simulink model "RoboticFish_NGC"  (R2020b)
settings: Solver=ode4  StartTime=0.0  StopTime=120  FixedStep=0.00025  RelTol=1e-3  EnableMultiTasking=on
undefined symbols (not defined in the file or in its folder): sigbuilder_block
undefined symbols (not defined in the file): Ref, uCMD
libraries: sharedutil x11, pid_lib x5, dspsigops x2, dspmtrx3 x1, vrlib x1
(part 1 of 2)
settings Model: Creator=Waqas Ali Waqar  LastModifiedBy=Waqas Ali Waqar
settings SolverCC: ConcurrentTasks=on  AutoInsertRateTranBlk=on  InsertRTBMode=Never (minimum delay)
settings DataIOCC: SaveFormat=StructureWithTime
settings OptimizationCC: BlockReduction=off  OptimizeBlockIOStorage=off  BufferReuse=off  GlobalBufferReuse=off  ExpressionFolding=off  PassReuseOutputArgsThreshold=0  LocalBlockOutputs=off  OptimizeBlockOrder=speed  OptimizeDataStoreBuffers=off  BusAssignmentInplaceUpdate=off
settings DebuggingCC: ParameterTunabilityLossMsg=error
settings HardwareCC: ProdBitPerPointer=32  ProdBitPerSizeT=32  ProdBitPerPtrDiffT=32  ProdLargestAtomicFloat=None  ProdWordSize=32  ProdLongLongMode=on  ProdHWDeviceType=Generic->32-bit x86 compatible
settings SFSimCC: MATLABDynamicMemAlloc=off  CustomCodeUndefinedFunction=UseInterfaceOnly
settings RTWCC: GenerateReport=on  RTWVerbose=off  LaunchReport=on  RTWCompilerOptimization=on
settings CodeAppCC: ForceParamTrailComments=on  OperatorAnnotations=on
settings GRTTargetCC: TargetLangStandard=C89/C90 (ANSI)

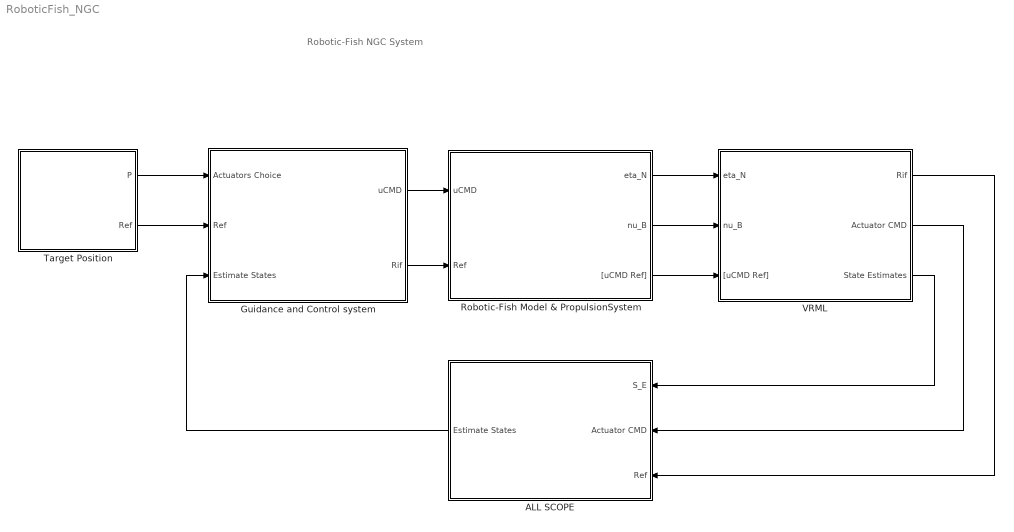
== system RoboticFish_NGC ==
  note: Robotic-Fish NGC System
  ALL SCOPE : Subsystem
  Guidance and Control system : Subsystem
  Robotic-Fish Model & PropulsionSystem : Subsystem  mask{Ig=[0.0268 0 0;0 0.0512 0;0 0 0.043], m=3.259, rho=1000, R=0.05, L=0.55, cdf=0.5, cdt=1, W=32.59, B=32.59, rG_B=[0;0;0], rB_B=[0;0;-0.02], DL=diag([0;0;0;0;0;0]), c=0.14, S=0.014, Theta0deg=15, a2=3.60, a1=-0.026, a0=-0.163, b2=8.952, b1=-0.359, b0=0.012, c2=51.81, d2=33.01, phisurge=0.59, phisway=0.44, phiyaw=0.53, cL=2, xfin=0.11, yfin=0.11, zfin=0.75, Max_Delta=45, Min_Delta=-45, Sfin=0.017, HT1Max=1.12, e1=[1;0;0], r1=[0;-0.11;0], HT2Max=1.12, e2=[1;0;0], r2=[0;0.11;0], VT1Max=1.12, e3=[0;0;1], r3=[0;0;-0.03]}
      mask prompts: Ig "Inertia Tensor Ig:"; m "Mass m:"; rho "Seawater Density rho:"; R "Body Radius R:"; L "Body Lenght L:"; cdf "Drag Weight cdf:"; cdt "Drag Weight cdt [0.8-1.2]:"; W "Weight"; B "Buoyancy"; DL "Linear Damping Matrix"; c "c-Foil Mean Chord (m)"; S "S-Foil area (m^2)"; Theta0deg "Theta0-Oscillation amplitude"; cL "fin lift coefficient  cL:"; xfin "fin axial position xfin:"; yfin "fin axial position yfin:"; zfin "fin axial position zfin:"; Max_Delta "Max fin rotation angle"; Min_Delta "Min fin rotation angle"; Sfin "fin platform area Sfin:"; HT1Max "Max Thrust (HT1):"; e1 "e1 (HT1):"; r1 "r1 (HT1):"; HT2Max "Max Thrust (HT2):"; e2 "e2 (HT2 ):"; r2 "r2 (HT2):"; VT1Max "Max Thrust (VT1):"; e3 "e3 (VT1):"; r3 "r3 (VT1):"
      mask init:
      | %%%%%%%%%%%%%%%%%%%%%%%%%%%%%%%%%%%%%%%%%%%%%%%%%%%%%%%
      | %%%%%%%%%%%%%%%%%%%  DINAMICA  %%%%%%%%%%%%%%%%%%%%%%%%
      | %%%%%%%%%%%%%%%%%%%%%%%%%%%%%%%%%%%%%%%%%%%%%%%%%%%%%%%
      | 
      | % Matrice di inerzia del corpo rigido
      | Ib = Ig-m*skewsymm(rG_B)*skewsymm(rG_B);
      | MRB = [m*eye(3,3) -m*skewsymm(rG_B); m*skewsymm(rG_B) Ib];
      | 
      | %Masse aggiunte
      | X_udot = 0.1*m;
      | Y_vdot = pi*rho*R^2*L;
      | Z_wdot = pi*rho*R^2*L;
      | K_pdot = 0;
      | M_qdot = (pi*rho*R^2*L^3)/12;
      | N_rdot = (pi*rho*R^2*L^3)/12;
      | 
      | %Matrice delle masse aggiunte
      | MA = diag([X_udot;Y_vdot;Z_wdot;K_pdot;M_qdot;N_rdot]);
      | 
      | %Matrice di inerzia (incluse le masse aggiunte)
      | M = MRB + MA;
      | inv_M = inv(M);
      | M11 = MA(1:3,1:3);    M12 = MA(1:3,4:6);
      | M21 = MA(4:6,1:3);    M22 = MA(4:6,4:6);
      | 
      | %%Attrito viscoso
      | 
      | %Aree
      | Af = pi*R^2;
      | At = 2*pi*R;
      | 
      | %Coefficienti
      | X_uu = 2*rho*Af*cdf/2;
      | Y_vv = rho*At*cdt/2;
      | Z_ww = rho*At*cdt/2;
      | K_pp = (rho*At*cdt*L^3)/16;
      | M_qq = (rho*At*cdt*L^3)/16;
      | N_rr = (rho*At*cdt*L^3)/16;
      | 
      | dQ = ([X_uu;Y_vv;Z_ww;K_pp;M_qq;N_rr]);
      | 
      | 
      | %%%%%%%%%%%%%%%%%%%%%%%%%%%%%%%%%%%%%%%%%%%%%%%%%%%%%%%
      | %%%%%%%%%%%%%%%%%%%  PROP HT3  %%%%%%%%%%%%%%%%%%%%%%%%
      | %%%%%%%%%%%%%%%%%%%%%%%%%%%%%%%%%%%%%%%%%%%%%%%%%%%%%%%
      | 
      | Theta0=Theta0deg*pi/180
      | TanTheta0=tan(Theta0)
      | 
      | 
      | %%%%%%%%%%%%%%%%%%%%%%%%%%%%%%%%%%%%%%%%%%%%%%%%%%%%%%%
      | %%%%%%%%%%%%%%%%%%%  PROP HT1 HT2 VT1  %%%%%%%%%%%%%%%%
      | %%%%%%%%%%%%%%%%%%%%%%%%%%%%%%%%%%%%%%%%%%%%%%%%%%%%%%%
      | 
      | K1 = HT1Max*9.81;
      | K2 = HT2Max*9.81;
      | K3 = VT1Max*9.81;
      | HT_prop = [e1 e2;skewsymm(r1)*e1 skewsymm(r2)*e2]*diag([K1;K2]);
      | VT_prop = [e3 ;skewsymm(r3)*e3 ]*K3;
      | 
      | 
      | %%%%%%%%%%%%%%%%%%%%%%%%%%%%%%%%%%%%%%%%%%%%%%%%%%%%%%%
      | %%%%%%%%%%%%%%%%%%%  PROP VT1 VT2  %%%%%%%%%%%%%%%%%%%%
      | %%%%%%%%%%%%%%%%%%%%%%%%%%%%%%%%%%%%%%%%%%%%%%%%%%%%%%%
      | 
      | Max_Delta_rad=Max_Delta*pi/180;
      | Min_Delta_rad=Min_Delta*pi/180;
      mask DialogControl DescGroupVar Prompt: Robotic Fish Paramteres
      mask DialogControl Container14 Prompt: Robotic Fish Parameters
      mask DialogControl Container17 Prompt: Caudal Fin Parameters
      mask DialogControl Container18 Prompt: Pectoral Fins Parameters
      mask DialogControl Container19 Prompt: Thrusters Parameters
  Target Position : Subsystem  mask{PC=Normal, SP=Way-Points based Path, Xr=0, Yr=0, Zr=0}
      mask init:
      | if (SP == 1)
      |     Flag=0;
      | end
      | if (SP == 2)
      |     Flag=1;
      | end
      | 
      | if (PC == 1)
      |     PropChoice=0;
      | end
      | if (PC == 2)
      |     PropChoice=1;
      | end
      mask TypeOptions PC: Normal | Only Propeller
      mask TypeOptions SP: Way-Points based Path | Way-Point Position
      mask DialogControl DescGroupVar Prompt: Target Position
      mask DialogControl Container8 Prompt: Actuator Choice
      mask DialogControl Container7 Prompt: Select Target
      mask DialogControl Container9 Prompt: Way-Point position
  "VRML " : Subsystem
  wires:
  Robotic-Fish Model & PropulsionSystem/2(nu_B) -> "VRML "/2(nu_B)
  Target Position/1(P) -> Guidance and Control system/1(Actuators Choice)
  Robotic-Fish Model & PropulsionSystem/1(eta_N) -> "VRML "/1(eta_N)
  Target Position/2(Ref) -> Guidance and Control system/2(Ref)
  ALL SCOPE/1(Estimate States) -> Guidance and Control system/3(Estimate States)
  "VRML "/3(State Estimates) -> ALL SCOPE/1(S_E)
  "VRML "/2(Actuator CMD) -> ALL SCOPE/2(Actuator CMD)
  "VRML "/1(Rif) -> ALL SCOPE/3(Ref)
  Robotic-Fish Model & PropulsionSystem/3("[uCMD Ref]") -> "VRML "/3("[uCMD Ref]")
  Guidance and Control system/1(uCMD) -> Robotic-Fish Model & PropulsionSystem/1(uCMD)
  Guidance and Control system/2(Rif) -> Robotic-Fish Model & PropulsionSystem/2(Ref)

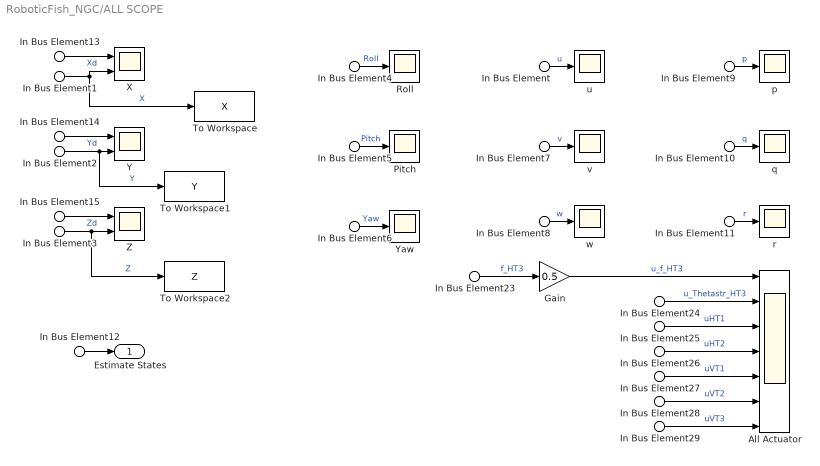
== system RoboticFish_NGC/ALL SCOPE ==
  In Bus Element12 : Inport  PortName=S_E
  In Bus Element2 : Inport  PortName=S_E  Element=Position.Y
  In Bus Element3 : Inport  PortName=S_E  Element=Position.Z
  In Bus Element4 : Inport  PortName=S_E  Element=Position.Roll
  In Bus Element5 : Inport  PortName=S_E  Element=Position.Pitch
  In Bus Element6 : Inport  PortName=S_E  Element=Position.Yaw
  In Bus Element1 : Inport  PortName=S_E  Element=Position.X
  In Bus Element : Inport  PortName=S_E  Element=Velocity.u
  In Bus Element7 : Inport  PortName=S_E  Element=Velocity.v
  In Bus Element8 : Inport  PortName=S_E  Element=Velocity.w
  In Bus Element9 : Inport  PortName=S_E  Element=Velocity.p
  In Bus Element10 : Inport  PortName=S_E  Element=Velocity.q
  In Bus Element11 : Inport  PortName=S_E  Element=Velocity.r
  In Bus Element23 : Inport  Port=2  PortName=Actuator CMD  Element=f_HT3
  In Bus Element24 : Inport  Port=2  PortName=Actuator CMD  Element=Thetastr_HT3
  In Bus Element25 : Inport  Port=2  PortName=Actuator CMD  Element=uHT1
  In Bus Element26 : Inport  Port=2  PortName=Actuator CMD  Element=uHT2
  In Bus Element27 : Inport  Port=2  PortName=Actuator CMD  Element=uVT1
  In Bus Element28 : Inport  Port=2  PortName=Actuator CMD  Element=D_VT2
  In Bus Element29 : Inport  Port=2  PortName=Actuator CMD  Element=D_VT3
  In Bus Element13 : Inport  Port=3  PortName=Ref  Element=Xr
  In Bus Element14 : Inport  Port=3  PortName=Ref  Element=Yr
  In Bus Element15 : Inport  Port=3  PortName=Ref  Element=Zr
  All Actuator : Scope  NumInputPorts=7
  Gain : Gain  Gain=0.5
  Pitch : Scope
  Roll : Scope
  To Workspace : ToWorkspace  VariableName=X  SampleTime=0.25
  To Workspace1 : ToWorkspace  VariableName=Y  SampleTime=0.25
  To Workspace2 : ToWorkspace  VariableName=Z  SampleTime=0.25
  X : Scope  NumInputPorts=2
  Y : Scope  NumInputPorts=2
  Yaw : Scope
  Z : Scope  NumInputPorts=2
  p : Scope
  q : Scope
  r : Scope
  u : Scope
  v : Scope
  w : Scope
  Estimate States : Outport  VectorParamsAs1DForOutWhenUnconnected=off
  wires:
  In Bus Element4/1 -> Roll/1  "Roll"
  In Bus Element5/1 -> Pitch/1  "Pitch"
  In Bus Element6/1 -> Yaw/1  "Yaw"
  In Bus Element/1 -> u/1  "u"
  In Bus Element7/1 -> v/1  "v"
  In Bus Element8/1 -> w/1  "w"
  In Bus Element9/1 -> p/1  "p"
  In Bus Element10/1 -> q/1  "q"
  In Bus Element11/1 -> r/1  "r"
  In Bus Element12/1 -> Estimate States/1
  In Bus Element15/1 -> Z/1  "Zd"
  In Bus Element3/1 -> To Workspace2/1, Z/2  "Z"
  In Bus Element2/1 -> To Workspace1/1, Y/2  "Y"
  In Bus Element14/1 -> Y/1  "Yd"
  In Bus Element23/1 -> Gain/1  "f_HT3"
  In Bus Element24/1 -> All Actuator/2  "u_Thetastr_HT3"
  In Bus Element25/1 -> All Actuator/3  "uHT1"
  In Bus Element26/1 -> All Actuator/4  "uHT2"
  In Bus Element27/1 -> All Actuator/5  "uVT1"
  In Bus Element28/1 -> All Actuator/6  "uVT2"
  In Bus Element29/1 -> All Actuator/7  "uVT3"
  Gain/1 -> All Actuator/1  "u_f_HT3"
  In Bus Element1/1 -> To Workspace/1, X/2  "X"
  In Bus Element13/1 -> X/1  "Xd"

== system RoboticFish_NGC/Guidance and Control system ==
  Actuators Choice : Inport
  Ref : Inport  Port=2
  Estimate States : Inport  Port=3
  " Control system" : Subsystem
  " Guidance system" : Subsystem
  uCMD : Outport  VectorParamsAs1DForOutWhenUnconnected=off
  Rif : Outport  Port=2  VectorParamsAs1DForOutWhenUnconnected=off
  wires:
  Estimate States/1 -> " Guidance system"/2(Estimate States I)
  Ref/1 -> Rif/1, " Guidance system"/1(Ref)
  " Guidance system"/1("LOS ") -> " Control system"/1(LOS)
  Actuators Choice/1 -> " Control system"/2(Actuators Choice)
  " Guidance system"/2(Estimate States O) -> " Control system"/3(Estimate states)
  " Control system"/1(uCMD) -> uCMD/1

== system RoboticFish_NGC/Robotic-Fish Model & PropulsionSystem ==
  uCMD : Inport
  In Bus Element1 : Inport  Port=2  PortName=Ref
  Bus Creator : BusCreator  Inputs=2
  Memory : Memory
  Propulsion System : Subsystem
  RF Dynamics and Kinematics (Attitude rappresentation: Quaternions) : Subsystem
      mask Display: image('C:\Users\Waqas Ali Waqar\Desktop\Robotic_Fish_Simulink\Robotic_Fish_Simulink\Imm\RF.png');
  eta_N : Outport  VectorParamsAs1DForOutWhenUnconnected=off
  nu_B : Outport  Port=2  VectorParamsAs1DForOutWhenUnconnected=off
  "[uCMD Ref]" : Outport  Port=3  VectorParamsAs1DForOutWhenUnconnected=off
  wires:
  RF Dynamics and Kinematics (Attitude rappresentation: Quaternions)/1(nu_B) -> nu_B/1, Memory/1  "[u    v    w    p    q    r]"
  Memory/1 -> Propulsion System/1(nu_B)
  RF Dynamics and Kinematics (Attitude rappresentation: Quaternions)/2(eta_N) -> eta_N/1  "[x   y   z  q0  q1  q2  q3]"
  uCMD/1 -> Propulsion System/2(uCMD)
  Propulsion System/2(ucmd) -> Bus Creator/1  "uCMD"
  Propulsion System/1(Tau_B) -> RF Dynamics and Kinematics (Attitude rappresentation: Quaternions)/1(tau_B)  "[Tau_X, Tau_Y, Tau_Z, Tau_Roll, Tau_Pitch, Tau_Yaw]"
  In Bus Element1/1 -> Bus Creator/2  "Ref"
  Bus Creator/1 -> "[uCMD Ref]"/1

== system RoboticFish_NGC/Target Position ==
  "  " : Subsystem  Tag=STV Subsys  LoadFcn=sigbuilder_block('load');  StartFcn=sigbuilder_block('start');  StopFcn=sigbuilder_block('stop');  ClipboardFcn=sigbuilder_block('clipboard');  mask(Sigbuilder block){tuvar=[0:10]}
      mask help: Simulink:masks:SigbuilderBlock_MD
      mask init:
      | if ~strcmp(get_param(bdroot(gcbh),'SimulationStatus'),'stopped') tuvar = sigbuilder_block('maskInit'); end
      settings: CopyFcn=sigbuilder_block('copy');  DeleteFcn=sigbuilder_block('delete');  ModelCloseFcn=sigbuilder_block('modelClose');  PreSaveFcn=sigbuilder_block('preSave');  PauseFcn=sigbuilder_block('pause');  ContinueFcn=sigbuilder_block('continue');  NameChangeFcn=sigbuilder_block('namechange');  OpenFcn=sigbuilder_block('open',[6 30 1012.5 447.75 ]);  CloseFcn=sigbuilder_block('close');
      mask Display: plot(0, 0, 100, 100,[2, 2, 32, 32, 2], [68, 8, 8, 68, 68],[32, 2], [38, 38], [32, 19, 2],[53, 60, 44], [32, 17, 17, 2],[16, 16, 31, 31]);txt = getActiveGroup(gcbh);text(2, 100, txt,'verticalAlignment', 'top');
  Bus Creator : BusCreator  Inputs=3
  Bus Creator1 : BusCreator  Inputs=3
  Constant : Constant  Value=Flag
  Constant1 : Constant  Value=Xr
  Constant2 : Constant  Value=Yr
  Constant3 : Constant  Value=Zr
  Constant4 : Constant  Value=PropChoice
  Switch : Switch  Criteria=u2 > Threshold
  Bus Element Out : Outport  VectorParamsAs1DForOutWhenUnconnected=off  PortName=P  Element=Actuators Choice
  Ref : Outport  Port=2  VectorParamsAs1DForOutWhenUnconnected=off
  wires:
  "  "/3(Zr) -> Bus Creator1/3  "Zr"
  Constant/1 -> Switch/2
  Bus Creator1/1 -> Switch/3
  Bus Creator/1 -> Switch/1
  Switch/1 -> Ref/1
  Constant3/1 -> Bus Creator/3  "Zr"
  Constant2/1 -> Bus Creator/2  "Yr"
  Constant1/1 -> Bus Creator/1  "Xr"
  Constant4/1 -> Bus Element Out/1  "PCHOICE"
  "  "/2(Yr) -> Bus Creator1/2  "Yr"
  "  "/1(Xr) -> Bus Creator1/1  "Xr"

== system RoboticFish_NGC/VRML  ==
  eta_N : Inport
  nu_B : Inport  Port=2
  In Bus Element1 : Inport  Port=3  PortName=[uCMD Ref]  Element=uCMD
  In Bus Element : Inport  Port=3  PortName=[uCMD Ref]  Element=Ref
  In Bus Element2 : Inport  Port=3  PortName=[uCMD Ref]  Element=Ref
  Bus Selector : BusSelector  OutputSignals=uVT3,uVT2,uHT3,uVT1,uHT2,uHT1
  Estimate States : Subsystem
  RF Position and Rotation to VR Translation and Rotation : Subsystem
  RF Virtual Reality Display : vrlib/VR Sink  InstantiateOnLoad=on  SampleTime=0.1  ViewEnable=on  RemoteChange=off  RemoteView=off  FieldsWritten=WayPoint.rotation.4.1.1.double#WayPoint.translation.3.1.1.double#RF.rotation.4.1.1.double#RF.translation.3.1.1.double#VT3.rotation.4.1.1.double#Vt2.rotation.4.1.1.double#HT3.rotation.4.1.1.double#VT1.rotation.4.1.1.double#HT2.rotation.4.1.1.double#HT1.rotation.4.1.1.double#ViewPoints.translation.3.1.1.double  WorldFileName=Final_RF.wrl  AutoView=on  VideoDimensions=[]  AllowVariableSize=off  FigureProperties="{'Position', 'Name', 'Viewpoint', 'CameraBound', 'CameraDirection', 'CameraPosition', 'CameraUpVector', 'ZoomFactor', 'Antialiasing', 'Headlight', 'Lighting', 'NavPanel', 'Sound', 'StatusBar', 'Stereo3D', 'Stereo3DCameraOffset', 'Stereo3DHIT', 'ToolBar', 'Textures', 'Transparency', 'Triad', 'Wireframe', 'NavZones', 'NavMode', 'NavSpeed', 'CaptureFileFormat', 'CaptureFileName', 'Record2DCompressMethod', 'Record2DCompressQuality', 'Record2D', 'Record2DFileName', 'Record2DFPS'; [5.0000000000000000e+00   1.2200000000000000e+02   5.7600000000000000e+02   3.2000000000000000e+02], '', 'RF_UP_CAMERA', 'on', [0.0000000000000000e+00   0.0000000000000000e+00  -1.0000000000000000e+00], [0.0000000000000000e+00   0.0000000000000000e+00   0.0000000000000000e+00], [0.0000000000000000e+00   1.0000000000000000e+00   0.0000000000000000e+00], [1.0000000000000000e+00], 'on', 'on', 'on', 'halfbar', 'on', 'on', 'off', [1.0000000149011612e-01], [0.0000000000000000e+00], 'on', 'on', 'on', 'none', 'off', 'off', 'fly', 'normal', 'tif', '%f_anim_%n.tif', 'auto', [7.5000000000000000e+01], 'off', '%f_anim_%n.avi', 'auto'}"
  Thruster rotation : Subsystem
  WayPoint Position and Rotation To VR Translation and Rotation : Subsystem
  Rif : Outport  VectorParamsAs1DForOutWhenUnconnected=off
  Actuator CMD : Outport  Port=2  VectorParamsAs1DForOutWhenUnconnected=off
  State Estimates : Outport  Port=3  VectorParamsAs1DForOutWhenUnconnected=off
  wires:
  eta_N/1 -> Estimate States/2(eta), RF Position and Rotation to VR Translation and Rotation/1(eta_N)
  nu_B/1 -> Estimate States/1(nu)
  RF Position and Rotation to VR Translation and Rotation/1(VR Rotation) -> WayPoint Position and Rotation To VR Translation and Rotation/2(RF VR Rotation), RF Virtual Reality Display/3
  Estimate States/1(Estimate States) -> State Estimates/1
  In Bus Element2/1 -> WayPoint Position and Rotation To VR Translation and Rotation/1(Waypoint Position)
  Thruster rotation/1(T_rotation) -> Bus Selector/1
  In Bus Element1/1 -> Actuator CMD/1, Thruster rotation/1(uCMD)
  In Bus Element/1 -> Rif/1
  WayPoint Position and Rotation To VR Translation and Rotation/2(Waypoint VR Translation) -> RF Virtual Reality Display/2
  WayPoint Position and Rotation To VR Translation and Rotation/1(Waypoint VR Rotation) -> RF Virtual Reality Display/1
  Bus Selector/1 -> RF Virtual Reality Display/5  "<uVT3>"
  Bus Selector/2 -> RF Virtual Reality Display/6  "<uVT2>"
  Bus Selector/3 -> RF Virtual Reality Display/7  "<uHT3>"
  Bus Selector/4 -> RF Virtual Reality Display/8  "<uVT1>"
  Bus Selector/5 -> RF Virtual Reality Display/9  "<uHT2>"
  Bus Selector/6 -> RF Virtual Reality Display/10  "<uHT1>"
  RF Position and Rotation to VR Translation and Rotation/2(VR Translation) -> RF Virtual Reality Display/11, RF Virtual Reality Display/4

== system RoboticFish_NGC/Guidance and Control system/ Control system ==
  LOS : Inport
  Actuators Choice : Inport  Port=2
  Estimate states : Inport  Port=3
  Control Allocator : Subsystem
  Control Law : Subsystem
  uCMD : Outport  VectorParamsAs1DForOutWhenUnconnected=off
  wires:
  Control Law/1(Tin) -> Control Allocator/1(Tin)
  LOS/1 -> Control Law/1(LOS)
  Estimate states/1 -> Control Law/2(Estimate States)
  Control Law/2(Actuators Choice O) -> Control Allocator/2(Actuators Choice)
  Control Allocator/1(uCMD) -> uCMD/1
  Actuators Choice/1 -> Control Law/3(P)

== system RoboticFish_NGC/Guidance and Control system/ Guidance system ==
  In Bus Element9 : Inport  PortName=Ref  Element=Xr
  In Bus Element10 : Inport  PortName=Ref  Element=Yr
  In Bus Element8 : Inport  PortName=Ref  Element=Zr
  In Bus Element3 : Inport  Port=2  PortName=Estimate States I
  In Bus Element4 : Inport  Port=2  PortName=Estimate States I  Element=Position.X
  In Bus Element5 : Inport  Port=2  PortName=Estimate States I  Element=Position.Y
  In Bus Element6 : Inport  Port=2  PortName=Estimate States I  Element=Position.Z
  Bus Creator : BusCreator  Inputs=3
  Distance : Subsystem
  LOS law : Subsystem
  Mux1 : Mux  Inputs=3
  Mux4 : Mux  Inputs=3
  Selector : Selector  InputPortWidth=3  IndexOptions=Index vector (dialog)  Indices=[3]  OutputSizes=1
  Selector1 : Selector  InputPortWidth=3  IndexOptions=Index vector (dialog)  Indices=[1 2]  OutputSizes=1
  Selector2 : Selector  InputPortWidth=3  IndexOptions=Index vector (dialog)  Indices=[1 2]  OutputSizes=1
  Sum2 : Sum  Inputs=|+-
  "LOS " : Outport  VectorParamsAs1DForOutWhenUnconnected=off
  Estimate States O : Outport  Port=2  VectorParamsAs1DForOutWhenUnconnected=off
  wires:
  In Bus Element3/1 -> Estimate States O/1
  In Bus Element4/1 -> Mux1/1
  In Bus Element5/1 -> Mux1/2
  LOS law/1(Yaw_d) -> Bus Creator/2  "Yaw_d"
  Selector/1 -> Bus Creator/3  "Ze"
  Bus Creator/1 -> "LOS "/1
  Sum2/1 -> Selector1/1, Selector/1, Selector2/1  "[Xe Ye Ze]"
  Distance/1(D) -> Bus Creator/1  "D"
  In Bus Element9/1 -> Mux4/1
  In Bus Element10/1 -> Mux4/2
  Mux4/1 -> Sum2/1  "[Xr Yr Zr]"
  Mux1/1 -> Sum2/2  "[X Y Z]"
  Selector1/1 -> Distance/1("[Xe Ye]")  "[Xe Ye]"
  Selector2/1 -> LOS law/1("[Xe Ye]")  "[Xe Ye]"
  In Bus Element6/1 -> Mux1/3
  In Bus Element8/1 -> Mux4/3

== system RoboticFish_NGC/Robotic-Fish Model & PropulsionSystem/Propulsion System ==
  nu_B : Inport
  In Bus Element : Inport  Port=2  PortName=uCMD
  In Bus Element1 : Inport  Port=2  PortName=uCMD  Element=f_HT3
  In Bus Element4 : Inport  Port=2  PortName=uCMD  Element=uHT2
  In Bus Element5 : Inport  Port=2  PortName=uCMD  Element=uVT1
  In Bus Element6 : Inport  Port=2  PortName=uCMD  Element=uVT2
  In Bus Element7 : Inport  Port=2  PortName=uCMD  Element=uVT3
  In Bus Element8 : Inport  Port=2  PortName=uCMD  Element=Thetastr_HT3
  In Bus Element2 : Inport  Port=2  PortName=uCMD  Element=uHT1
  Bus Creator : BusCreator  Inputs=2
  Bus Creator1 : BusCreator  Inputs=2
  Horizontal Force and Moment (Tau_H) : Subsystem
  Subsystem : Subsystem
  Sum : Sum  Inputs=|++
  Vertical Force and Moment (Tau_V) : Subsystem
  Tau_B : Outport  VectorParamsAs1DForOutWhenUnconnected=off
  ucmd : Outport  Port=2  VectorParamsAs1DForOutWhenUnconnected=off
  wires:
  nu_B/1 -> Horizontal Force and Moment (Tau_H)/4(nu_B), Vertical Force and Moment (Tau_V)/1(nu_B)
  Sum/1 -> Tau_B/1  "Horizontal_Tau+Vertical_Tau"
  Horizontal Force and Moment (Tau_H)/1(Horizontal _Tau) -> Sum/1
  Vertical Force and Moment (Tau_V)/1(Vertical_Tau) -> Sum/2
  In Bus Element6/1 -> Bus Creator/1
  In Bus Element7/1 -> Bus Creator/2
  Bus Creator/1 -> Vertical Force and Moment (Tau_V)/3("[uVT2 uVT3]")
  In Bus Element5/1 -> Vertical Force and Moment (Tau_V)/2(uVT1)
  In Bus Element4/1 -> Horizontal Force and Moment (Tau_H)/3(uHT2)
  In Bus Element2/1 -> Horizontal Force and Moment (Tau_H)/2(uHT1)
  In Bus Element1/1 -> Bus Creator1/1
  In Bus Element8/1 -> Bus Creator1/2
  Bus Creator1/1 -> Horizontal Force and Moment (Tau_H)/1(uHT3)
  Vertical Force and Moment (Tau_V)/2("[Delta_VT2 Delta_VT3]") -> Subsystem/1(D_uVT2  D_uVT3)
  In Bus Element/1 -> Subsystem/2(uCMD)
  Subsystem/1("ucmd ") -> ucmd/1

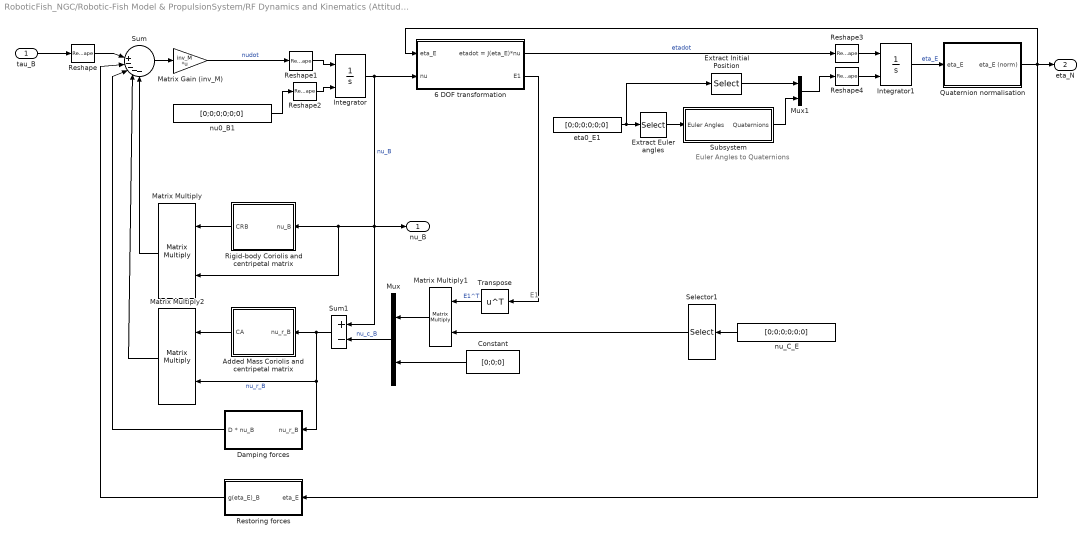
== system RoboticFish_NGC/Robotic-Fish Model & PropulsionSystem/RF Dynamics and Kinematics (Attitude rappresentation: Quaternions) ==
  note: E1
  note: Euler Angles to Quaternions
  tau_B : Inport
  6 DOF transformation : Subsystem  AncestorBlock=MarineGNC/Library blocks/Axes transformations/6 DOF transformation
  Added Mass Coriolis and centripetal matrix : Subsystem
  Constant : Constant  Value=[0;0;0]
  Damping forces : Subsystem
  Extract Euler angles : Selector  InputPortWidth=6  IndexOptions=Index vector (dialog)  Indices=[4 5 6]  OutputSizes=1
  Extract Initial Position : Selector  InputPortWidth=6  IndexOptions=Index vector (dialog)  Indices=[1 2 3]  OutputSizes=1
  Integrator : Integrator  InitialConditionSource=external
  Integrator1 : Integrator  InitialConditionSource=external
  Matrix Gain (inv_M) : Gain  Gain=inv_M  Multiplication=Matrix(K*u)  SaturateOnIntegerOverflow=on  OutDataTypeStr=Inherit: Same as input  ParamDataTypeStr=Inherit: Same as input
  Matrix Multiply : Product  Multiplication=Matrix(*)
  Matrix Multiply1 : Product  Multiplication=Matrix(*)
  Matrix Multiply2 : Product  Multiplication=Matrix(*)
  Mux : Mux  Inputs=2
  Mux1 : Mux  Inputs=2
  Quaternion normalisation : Subsystem
  Reshape{,1..4} (5 alike) : Reshape  OutputDimensionality=Column vector (2-D)
  Restoring forces : Subsystem
  Rigid-body Coriolis and centripetal matrix : Subsystem
  Selector1 : Selector  InputPortWidth=6  IndexOptions=Index vector (dialog)  Indices=[1 2 3]  OutputSizes=1
  Subsystem : Subsystem
  Sum : Sum  Inputs=|||+----  SaturateOnIntegerOverflow=on
  Sum1 : Sum  Inputs=+-
  Transpose : Math  Operator=transpose  SignedPower=on  SaturateOnIntegerOverflow=on
  eta0_E1 : Constant  Value=[0;0;0;0;0;0]
  nu0_B1 : Constant  Value=[0;0;0;0;0;0]
  nu_C_E : Constant  Value=[0;0;0;0;0;0]
  nu_B : Outport  VectorParamsAs1DForOutWhenUnconnected=off
  eta_N : Outport  Port=2  VectorParamsAs1DForOutWhenUnconnected=off
  wires:
  Subsystem/1(Quaternions) -> Mux1/2
  Restoring forces/1(g(eta_E)_B) -> Sum/2
  eta0_E1/1 -> Extract Euler angles/1, Extract Initial Position/1
  Extract Initial Position/1 -> Mux1/1
  Selector1/1 -> Matrix Multiply1/2
  Matrix Gain (inv_M)/1 -> Reshape1/1  "nudot"
  Reshape4/1 -> Integrator1/2
  tau_B/1 -> Reshape/1
  Constant/1 -> Mux/2
  Quaternion normalisation/1(eta_E (norm)) -> 6 DOF transformation/1(eta_E), eta_N/1, Restoring forces/1(eta_E)
  Mux1/1 -> Reshape4/1
  nu_C_E/1 -> Selector1/1
  Extract Euler angles/1 -> Subsystem/1("Euler Angles ")
  Reshape/1 -> Sum/1
  Reshape1/1 -> Integrator/1
  Damping forces/1(D * nu_B) -> Sum/3
  Integrator1/1 -> Quaternion normalisation/1(eta_E)  "eta_E"
  6 DOF transformation/2(E1) -> Transpose/1
  Sum/1 -> Matrix Gain (inv_M)/1
  Rigid-body Coriolis and centripetal matrix/1(CRB) -> Matrix Multiply/1
  Mux/1 -> Sum1/2  "nu_c_B"
  6 DOF transformation/1(etadot = J(eta_E)*nu) -> Reshape3/1  "etadot"
  Integrator/1 -> 6 DOF transformation/2(nu), nu_B/1, Sum1/1, Rigid-body Coriolis and centripetal matrix/1(nu_B), Matrix Multiply/2  "nu_B"
  Matrix Multiply/1 -> Sum/5
  Transpose/1 -> Matrix Multiply1/1  "E1^T"
  Matrix Multiply1/1 -> Mux/1
  Sum1/1 -> Damping forces/1(nu_r_B), Matrix Multiply2/2, Added Mass Coriolis and centripetal matrix/1(nu_r_B)  "nu_r_B"
  nu0_B1/1 -> Reshape2/1
  Added Mass Coriolis and centripetal matrix/1(CA) -> Matrix Multiply2/1
  Reshape2/1 -> Integrator/2
  Matrix Multiply2/1 -> Sum/4
  Reshape3/1 -> Integrator1/1

== system RoboticFish_NGC/Target Position/   ==
  Demux : Demux  Tag=STV Demux  Outputs=3
      settings: DisplayOption=none
  FromWs : FromWorkspace  Tag=STV FromWs  VariableName=tuvar
      SigBuilderData=|
      | common.afterFinalStr = 'Extrapolate'
      | common.sampleTime = 0
      | dataSet.timeRange = [0 450]
      | dataSet.name = 'Waypoints generator'
      | sbobj.Groups.Name = 'Waypoints generator'
      | sbobj.Groups.Signals(1).Name = 'Xr'
      | sbobj.Groups.Signals(1).XData = [0 20 20 60 60 133.5 140 450]
      | sbobj.Groups.Signals(1).YData = [0 0 5 5 0 0 0 0]
      | sbobj.Groups.Signals(2).Name = 'Yr'
      | sbobj.Groups.Signals(2).XData = [0 14.5 20 40 40 80 80 450]
      | sbobj.Groups.Signals(2).YData = [0 0 0 0 5 5 0 0]
      | sbobj.Groups.Signals(3).Name = 'Zr'
      | sbobj.Groups.Signals(3).XData = [0 20 20 40 40 60 60 80 80 450]
      | sbobj.Groups.Signals(3).YData = [0 0 2 2 4 4 6 6 8 8]
      | sbobj.Groups.TimeRange = [0 450]
  Xr : Outport  Tag=STV Outport  VectorParamsAs1DForOutWhenUnconnected=off
  Yr : Outport  Tag=STV Outport  Port=2  VectorParamsAs1DForOutWhenUnconnected=off
  Zr : Outport  Tag=STV Outport  Port=3  VectorParamsAs1DForOutWhenUnconnected=off
  wires:
  FromWs/1 -> Demux/1
  Demux/1 -> Xr/1
  Demux/2 -> Yr/1
  Demux/3 -> Zr/1

== system RoboticFish_NGC/VRML /Estimate States ==
  nu : Inport
  eta : Inport  Port=2
  Gain : Gain  Gain=180/pi
  Mux : Mux  Inputs=2
  Quaternions to Euler Angles : Subsystem
  Subsystem : Subsystem
  eta1_E=[x,y,z]1 : Selector  InputPortWidth=7  IndexOptions=Index vector (dialog)  Indices=[1 2 3]  OutputSizes=1
  eta2_E=[q0,q1,q2,q3] : Selector  InputPortWidth=7  IndexOptions=Index vector (dialog)  Indices=[4 5 6 7]  OutputSizes=1
  Estimate States : Outport  VectorParamsAs1DForOutWhenUnconnected=off
  wires:
  eta2_E=[q0,q1,q2,q3]/1 -> Quaternions to Euler Angles/1(Quaternions)
  Mux/1 -> Subsystem/1(Position)
  eta1_E=[x,y,z]1/1 -> Mux/1
  eta/1 -> eta2_E=[q0,q1,q2,q3]/1, eta1_E=[x,y,z]1/1
  Subsystem/1(State Estimate) -> Estimate States/1
  Quaternions to Euler Angles/1(Euler Angles) -> Gain/1
  nu/1 -> Subsystem/2(nu_B)
  Gain/1 -> Mux/2

== system RoboticFish_NGC/VRML /RF Position and Rotation to VR Translation and Rotation ==
  eta_N : Inport
  Orientation to VR Rotation : Subsystem
  Position to VR Translation : Subsystem
  eta1_N=[x,y,z] : Selector  InputPortWidth=7  IndexOptions=Index vector (dialog)  Indices=[1 2 3]  OutputSizes=1
  eta2_N=[q0,q1,q2,q3] : Selector  InputPortWidth=7  IndexOptions=Index vector (dialog)  Indices=[4 5 6 7]  OutputSizes=1
  VR Rotation : Outport  VectorParamsAs1DForOutWhenUnconnected=off
  VR Translation : Outport  Port=2  VectorParamsAs1DForOutWhenUnconnected=off
  wires:
  eta2_N=[q0,q1,q2,q3]/1 -> Orientation to VR Rotation/1(Orientation)
  eta1_N=[x,y,z]/1 -> Position to VR Translation/1(Position)
  eta_N/1 -> eta1_N=[x,y,z]/1, eta2_N=[q0,q1,q2,q3]/1
  Orientation to VR Rotation/1(VR Rotation) -> VR Rotation/1
  Position to VR Translation/1(VR Translation) -> VR Translation/1

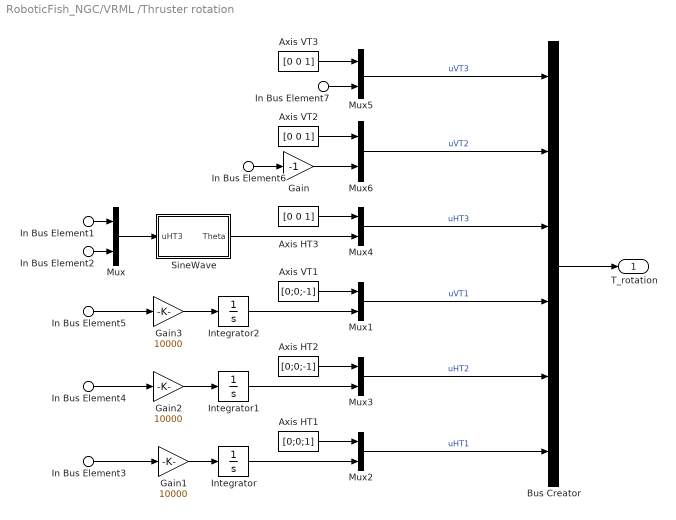
== system RoboticFish_NGC/VRML /Thruster rotation ==
  In Bus Element1 : Inport  PortName=uCMD  Element=f_HT3
  In Bus Element2 : Inport  PortName=uCMD  Element=Thetastr_HT3
  In Bus Element3 : Inport  PortName=uCMD  Element=uHT1
  In Bus Element4 : Inport  PortName=uCMD  Element=uHT2
  In Bus Element5 : Inport  PortName=uCMD  Element=uVT1
  In Bus Element6 : Inport  PortName=uCMD  Element=D_VT2
  In Bus Element7 : Inport  PortName=uCMD  Element=D_VT3
  Axis HT1 : Constant  Value=[0;0;1]
  Axis HT2 : Constant  Value=[0;0;-1]
  Axis HT3 : Constant  Value=[0 0 1]
  Axis VT1 : Constant  Value=[0;0;-1]
  Axis VT2 : Constant  Value=[0 0 1]
  Axis VT3 : Constant  Value=[0 0 1]
  Bus Creator : BusCreator  Inputs=6
  Gain : Gain  Gain=-1
  Gain1 : Gain  Gain=10000
  Gain2 : Gain  Gain=10000
  Gain3 : Gain  Gain=10000
  Integrator : Integrator
  Integrator1 : Integrator
  Integrator2 : Integrator
  Mux{,1..6} (7 alike) : Mux  Inputs=2
  SineWave : Subsystem  mask{Theta0=15}
      mask prompts: Theta0 "Theta0(Degrees)"
      mask init:
      | radTheta0=Theta0*pi/180
  T_rotation : Outport  VectorParamsAs1DForOutWhenUnconnected=off
  wires:
  Gain1/1 -> Integrator/1
  Axis HT3/1 -> Mux4/1
  Integrator1/1 -> Mux3/2
  Axis HT2/1 -> Mux3/1
  Integrator/1 -> Mux2/2
  SineWave/1(Theta) -> Mux4/2
  Integrator2/1 -> Mux1/2
  Axis VT1/1 -> Mux1/1
  Axis VT3/1 -> Mux5/1
  Axis VT2/1 -> Mux6/1
  Gain/1 -> Mux6/2
  Mux5/1 -> Bus Creator/1  "uVT3"
  Mux6/1 -> Bus Creator/2  "uVT2"
  Mux4/1 -> Bus Creator/3  "uHT3"
  Mux1/1 -> Bus Creator/4  "uVT1"
  Mux3/1 -> Bus Creator/5  "uHT2"
  Mux2/1 -> Bus Creator/6  "uHT1"
  Bus Creator/1 -> T_rotation/1
  In Bus Element7/1 -> Mux5/2
  In Bus Element6/1 -> Gain/1
  In Bus Element1/1 -> Mux/1
  In Bus Element2/1 -> Mux/2
  Mux/1 -> SineWave/1(uHT3)
  In Bus Element3/1 -> Gain1/1
  Gain2/1 -> Integrator1/1
  In Bus Element4/1 -> Gain2/1
  In Bus Element5/1 -> Gain3/1
  Gain3/1 -> Integrator2/1
  Axis HT1/1 -> Mux2/1

== system RoboticFish_NGC/VRML /WayPoint Position and Rotation To VR Translation and Rotation ==
  Waypoint Position : Inport
  RF VR Rotation : Inport  Port=2
  Way point Position to VR Translation : Subsystem
  Waypoint VR Rotation : Outport  VectorParamsAs1DForOutWhenUnconnected=off
  Waypoint VR Translation : Outport  Port=2  VectorParamsAs1DForOutWhenUnconnected=off
  wires:
  Way point Position to VR Translation/1(VR Translation) -> Waypoint VR Translation/1
  Waypoint Position/1 -> Way point Position to VR Translation/1(Position)
  RF VR Rotation/1 -> Waypoint VR Rotation/1

== system RoboticFish_NGC/Guidance and Control system/ Control system/Control Allocator ==
  Tin : Inport
  Actuators Choice : Inport  Port=2
  Matrix Multiply : Product  Multiplication=Matrix(*)
  Pseudoinverse choice : Subsystem
  Saturation limits : Subsystem
  uCMD : Outport  VectorParamsAs1DForOutWhenUnconnected=off
  wires:
  Saturation limits/1(uCMD) -> uCMD/1  "f_HT3 Thetastr_HT3  uHT1  uHT2  uVT1  uVT2  uVT3"
  Pseudoinverse choice/1(Pseudoinverse) -> Matrix Multiply/1
  Tin/1 -> Matrix Multiply/2, Pseudoinverse choice/1(Tin)  "[TX TN TZ]"
  Matrix Multiply/1 -> Saturation limits/1(InBus)  "f_HT3 Thetastr_HT3  uHT1  uHT2  uVT2  uVT3  uVT1"
  Actuators Choice/1 -> Pseudoinverse choice/2(Actuators Choice)

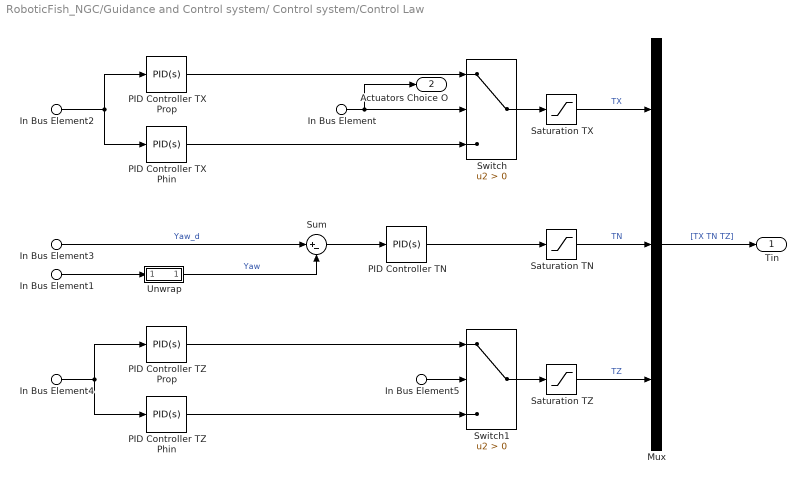
== system RoboticFish_NGC/Guidance and Control system/ Control system/Control Law ==
  In Bus Element2 : Inport  PortName=LOS  Element=D
  In Bus Element3 : Inport  PortName=LOS  Element=Yaw_d
  In Bus Element4 : Inport  PortName=LOS  Element=Ze
  In Bus Element1 : Inport  Port=2  PortName=Estimate States  Element=Position.Yaw
  In Bus Element : Inport  Port=3  PortName=P  Element=Actuators Choice
  In Bus Element5 : Inport  Port=3  PortName=P  Element=Actuators Choice
  Mux : Mux  Inputs=3
  PID Controller TN : pid_lib/PID Controller  Controller=PID  Form=Parallel  TimeDomain=Continuous-time  UseExternalTs=off  SampleTime=-1  IntegratorMethod=Forward Euler  FilterMethod=Forward Euler  ControllerParametersSource=internal  P=2  I=0  D=1  UseFilter=on  N=100  TunerSelectOption=Transfer Function Based (PID Tuner App)  InitialConditionSource=internal  InitialConditionForIntegrator=0  InitialConditionForFilter=0  DifferentiatorICPrevScaledInput=0  ExternalReset=none  TrackingMode=off  Kt=1  LimitOutput=off  SatLimitsSource=internal  UpperSaturationLimit=inf  LowerSaturationLimit=-inf  LinearizeAsGain=on  AntiWindupMode=none  Kb=1  POutMin=[]  POutMax=[]  IOutMin=[]  IOutMax=[]  DOutMin=[]  DOutMax=[]  NOutMin=[]  NOutMax=[]  SumOutMin=[]  SumOutMax=[]  SaturationOutMin=[]  SaturationOutMax=[]  PParamMin=[]  PParamMax=[]  IParamMin=[]  IParamMax=[]  DParamMin=[]  DParamMax=[]  NParamMin=[]  NParamMax=[]  KbParamMin=[]  KbParamMax=[]  KtParamMin=[]  KtParamMax=[]  KbOutMin=[]  KbOutMax=[]  KtOutMin=[]  KtOutMax=[]  IntegratorOutMin=[]  IntegratorOutMax=[]  FilterOutMin=[]  FilterOutMax=[]  SumI1OutMin=[]  SumI1OutMax=[]  SumI2OutMin=[]  SumI2OutMax=[]  SumI3OutMin=[]  SumI3OutMax=[]  SumI4OutMin=[]  SumI4OutMax=[]  SumDOutMin=[]  SumDOutMax=[]  DifferentiatorOutMin=[]  DifferentiatorOutMax=[]  FilterDiffOutCoefMin=[]  FilterDiffOutCoefMax=[]  ReciprocalOutMin=[]  ReciprocalOutMax=[]  SumDenOutMin=[]  SumDenOutMax=[]  SumNumOutMin=[]  SumNumOutMax=[]  DivideOutMin=[]  DivideOutMax=[]  UdiffTsProdOutMin=[]  UdiffTsProdOutMax=[]  NTsProdOutMin=[]  NTsProdOutMax=[]  UintegralTsProdOutMin=[]  UintegralTsProdOutMax=[]  UngainTsProdOutMin=[]  UngainTsProdOutMax=[]  IntegratorContinuousStateAttributes=''  IntegratorStateMustResolveToSignalObject=off  IntegratorRTWStateStorageClass=Auto  FilterContinuousStateAttributes=''  FilterStateMustResolveToSignalObject=off  FilterRTWStateStorageClass=Auto  ParallelPVariant=InternalParameters  IdealPVariant=Disabled  IVariant=InternalParameters  DVariant=InternalParameters  IntegratorVariant=Continuous  SatVariant=Disabled  AWVariant=Passthrough  PCopyVariant=Disabled  TRVariant=Disabled  FdbkBlocksVariant=Forward  IdealPFdbkVariant=Disabled  SatFdbkVariant=Disabled  DerivativeFilterVariant=ContFilter  NVariant=InternalParameters  NCopyVariant=Disabled  FilterICVariant=InternalICsFilter  IntegratorICVariant=InternalICs  ExternalResetVariant=Disabled  TRSumVariant=Passthrough  SumFdbkVariant=Disabled  SumVariant=Sum_PID  TsampFilterVariant=InternalTs  TsampNgainVariant=Passthrough  TsampIntegralVariant=Passthrough  ExternalSaturationOutDataTypeStr=Inherit: Same as second input
  PID Controller TX Phin : pid_lib/PID Controller  Controller=PID  Form=Parallel  TimeDomain=Continuous-time  UseExternalTs=off  SampleTime=-1  IntegratorMethod=Forward Euler  FilterMethod=Forward Euler  ControllerParametersSource=internal  P=1  I=0  D=0.2695  UseFilter=on  N=100  TunerSelectOption=Transfer Function Based (PID Tuner App)  InitialConditionSource=internal  InitialConditionForIntegrator=0  InitialConditionForFilter=0  DifferentiatorICPrevScaledInput=0  ExternalReset=none  TrackingMode=off  Kt=1  LimitOutput=off  SatLimitsSource=internal  UpperSaturationLimit=inf  LowerSaturationLimit=-inf  LinearizeAsGain=on  AntiWindupMode=none  Kb=1  POutMin=[]  POutMax=[]  IOutMin=[]  IOutMax=[]  DOutMin=[]  DOutMax=[]  NOutMin=[]  NOutMax=[]  SumOutMin=[]  SumOutMax=[]  SaturationOutMin=[]  SaturationOutMax=[]  PParamMin=[]  PParamMax=[]  IParamMin=[]  IParamMax=[]  DParamMin=[]  DParamMax=[]  NParamMin=[]  NParamMax=[]  KbParamMin=[]  KbParamMax=[]  KtParamMin=[]  KtParamMax=[]  KbOutMin=[]  KbOutMax=[]  KtOutMin=[]  KtOutMax=[]  IntegratorOutMin=[]  IntegratorOutMax=[]  FilterOutMin=[]  FilterOutMax=[]  SumI1OutMin=[]  SumI1OutMax=[]  SumI2OutMin=[]  SumI2OutMax=[]  SumI3OutMin=[]  SumI3OutMax=[]  SumI4OutMin=[]  SumI4OutMax=[]  SumDOutMin=[]  SumDOutMax=[]  DifferentiatorOutMin=[]  DifferentiatorOutMax=[]  FilterDiffOutCoefMin=[]  FilterDiffOutCoefMax=[]  ReciprocalOutMin=[]  ReciprocalOutMax=[]  SumDenOutMin=[]  SumDenOutMax=[]  SumNumOutMin=[]  SumNumOutMax=[]  DivideOutMin=[]  DivideOutMax=[]  UdiffTsProdOutMin=[]  UdiffTsProdOutMax=[]  NTsProdOutMin=[]  NTsProdOutMax=[]  UintegralTsProdOutMin=[]  UintegralTsProdOutMax=[]  UngainTsProdOutMin=[]  UngainTsProdOutMax=[]  IntegratorContinuousStateAttributes=''  IntegratorStateMustResolveToSignalObject=off  IntegratorRTWStateStorageClass=Auto  FilterContinuousStateAttributes=''  FilterStateMustResolveToSignalObject=off  FilterRTWStateStorageClass=Auto  ParallelPVariant=InternalParameters  IdealPVariant=Disabled  IVariant=InternalParameters  DVariant=InternalParameters  IntegratorVariant=Continuous  SatVariant=Disabled  AWVariant=Passthrough  PCopyVariant=Disabled  TRVariant=Disabled  FdbkBlocksVariant=Forward  IdealPFdbkVariant=Disabled  SatFdbkVariant=Disabled  DerivativeFilterVariant=ContFilter  NVariant=InternalParameters  NCopyVariant=Disabled  FilterICVariant=InternalICsFilter  IntegratorICVariant=InternalICs  ExternalResetVariant=Disabled  TRSumVariant=Passthrough  SumFdbkVariant=Disabled  SumVariant=Sum_PID  TsampFilterVariant=InternalTs  TsampNgainVariant=Passthrough  TsampIntegralVariant=Passthrough  ExternalSaturationOutDataTypeStr=Inherit: Same as second input
  PID Controller TX Prop : pid_lib/PID Controller  Controller=PID  Form=Parallel  TimeDomain=Continuous-time  UseExternalTs=off  SampleTime=-1  IntegratorMethod=Forward Euler  FilterMethod=Forward Euler  ControllerParametersSource=internal  P=1  I=0  D=1.2  UseFilter=on  N=100  TunerSelectOption=Transfer Function Based (PID Tuner App)  InitialConditionSource=internal  InitialConditionForIntegrator=0  InitialConditionForFilter=0  DifferentiatorICPrevScaledInput=0  ExternalReset=none  TrackingMode=off  Kt=1  LimitOutput=off  SatLimitsSource=internal  UpperSaturationLimit=inf  LowerSaturationLimit=-inf  LinearizeAsGain=on  AntiWindupMode=none  Kb=1  POutMin=[]  POutMax=[]  IOutMin=[]  IOutMax=[]  DOutMin=[]  DOutMax=[]  NOutMin=[]  NOutMax=[]  SumOutMin=[]  SumOutMax=[]  SaturationOutMin=[]  SaturationOutMax=[]  PParamMin=[]  PParamMax=[]  IParamMin=[]  IParamMax=[]  DParamMin=[]  DParamMax=[]  NParamMin=[]  NParamMax=[]  KbParamMin=[]  KbParamMax=[]  KtParamMin=[]  KtParamMax=[]  KbOutMin=[]  KbOutMax=[]  KtOutMin=[]  KtOutMax=[]  IntegratorOutMin=[]  IntegratorOutMax=[]  FilterOutMin=[]  FilterOutMax=[]  SumI1OutMin=[]  SumI1OutMax=[]  SumI2OutMin=[]  SumI2OutMax=[]  SumI3OutMin=[]  SumI3OutMax=[]  SumI4OutMin=[]  SumI4OutMax=[]  SumDOutMin=[]  SumDOutMax=[]  DifferentiatorOutMin=[]  DifferentiatorOutMax=[]  FilterDiffOutCoefMin=[]  FilterDiffOutCoefMax=[]  ReciprocalOutMin=[]  ReciprocalOutMax=[]  SumDenOutMin=[]  SumDenOutMax=[]  SumNumOutMin=[]  SumNumOutMax=[]  DivideOutMin=[]  DivideOutMax=[]  UdiffTsProdOutMin=[]  UdiffTsProdOutMax=[]  NTsProdOutMin=[]  NTsProdOutMax=[]  UintegralTsProdOutMin=[]  UintegralTsProdOutMax=[]  UngainTsProdOutMin=[]  UngainTsProdOutMax=[]  IntegratorContinuousStateAttributes=''  IntegratorStateMustResolveToSignalObject=off  IntegratorRTWStateStorageClass=Auto  FilterContinuousStateAttributes=''  FilterStateMustResolveToSignalObject=off  FilterRTWStateStorageClass=Auto  ParallelPVariant=InternalParameters  IdealPVariant=Disabled  IVariant=InternalParameters  DVariant=InternalParameters  IntegratorVariant=Continuous  SatVariant=Disabled  AWVariant=Passthrough  PCopyVariant=Disabled  TRVariant=Disabled  FdbkBlocksVariant=Forward  IdealPFdbkVariant=Disabled  SatFdbkVariant=Disabled  DerivativeFilterVariant=ContFilter  NVariant=InternalParameters  NCopyVariant=Disabled  FilterICVariant=InternalICsFilter  IntegratorICVariant=InternalICs  ExternalResetVariant=Disabled  TRSumVariant=Passthrough  SumFdbkVariant=Disabled  SumVariant=Sum_PID  TsampFilterVariant=InternalTs  TsampNgainVariant=Passthrough  TsampIntegralVariant=Passthrough  ExternalSaturationOutDataTypeStr=Inherit: Same as second input
  PID Controller TZ Phin : pid_lib/PID Controller  Controller=PID  Form=Parallel  TimeDomain=Continuous-time  UseExternalTs=off  SampleTime=-1  IntegratorMethod=Forward Euler  FilterMethod=Forward Euler  ControllerParametersSource=internal  P=0.6  I=0  D=0.6  UseFilter=on  N=100  TunerSelectOption=Transfer Function Based (PID Tuner App)  InitialConditionSource=internal  InitialConditionForIntegrator=0  InitialConditionForFilter=0  DifferentiatorICPrevScaledInput=0  ExternalReset=none  TrackingMode=off  Kt=1  LimitOutput=off  SatLimitsSource=internal  UpperSaturationLimit=inf  LowerSaturationLimit=-inf  LinearizeAsGain=on  AntiWindupMode=none  Kb=1  POutMin=[]  POutMax=[]  IOutMin=[]  IOutMax=[]  DOutMin=[]  DOutMax=[]  NOutMin=[]  NOutMax=[]  SumOutMin=[]  SumOutMax=[]  SaturationOutMin=[]  SaturationOutMax=[]  PParamMin=[]  PParamMax=[]  IParamMin=[]  IParamMax=[]  DParamMin=[]  DParamMax=[]  NParamMin=[]  NParamMax=[]  KbParamMin=[]  KbParamMax=[]  KtParamMin=[]  KtParamMax=[]  KbOutMin=[]  KbOutMax=[]  KtOutMin=[]  KtOutMax=[]  IntegratorOutMin=[]  IntegratorOutMax=[]  FilterOutMin=[]  FilterOutMax=[]  SumI1OutMin=[]  SumI1OutMax=[]  SumI2OutMin=[]  SumI2OutMax=[]  SumI3OutMin=[]  SumI3OutMax=[]  SumI4OutMin=[]  SumI4OutMax=[]  SumDOutMin=[]  SumDOutMax=[]  DifferentiatorOutMin=[]  DifferentiatorOutMax=[]  FilterDiffOutCoefMin=[]  FilterDiffOutCoefMax=[]  ReciprocalOutMin=[]  ReciprocalOutMax=[]  SumDenOutMin=[]  SumDenOutMax=[]  SumNumOutMin=[]  SumNumOutMax=[]  DivideOutMin=[]  DivideOutMax=[]  UdiffTsProdOutMin=[]  UdiffTsProdOutMax=[]  NTsProdOutMin=[]  NTsProdOutMax=[]  UintegralTsProdOutMin=[]  UintegralTsProdOutMax=[]  UngainTsProdOutMin=[]  UngainTsProdOutMax=[]  IntegratorContinuousStateAttributes=''  IntegratorStateMustResolveToSignalObject=off  IntegratorRTWStateStorageClass=Auto  FilterContinuousStateAttributes=''  FilterStateMustResolveToSignalObject=off  FilterRTWStateStorageClass=Auto  ParallelPVariant=InternalParameters  IdealPVariant=Disabled  IVariant=InternalParameters  DVariant=InternalParameters  IntegratorVariant=Continuous  SatVariant=Disabled  AWVariant=Passthrough  PCopyVariant=Disabled  TRVariant=Disabled  FdbkBlocksVariant=Forward  IdealPFdbkVariant=Disabled  SatFdbkVariant=Disabled  DerivativeFilterVariant=ContFilter  NVariant=InternalParameters  NCopyVariant=Disabled  FilterICVariant=InternalICsFilter  IntegratorICVariant=InternalICs  ExternalResetVariant=Disabled  TRSumVariant=Passthrough  SumFdbkVariant=Disabled  SumVariant=Sum_PID  TsampFilterVariant=InternalTs  TsampNgainVariant=Passthrough  TsampIntegralVariant=Passthrough  ExternalSaturationOutDataTypeStr=Inherit: Same as second input
  PID Controller TZ Prop : pid_lib/PID Controller  Controller=PID  Form=Parallel  TimeDomain=Continuous-time  UseExternalTs=off  SampleTime=-1  IntegratorMethod=Forward Euler  FilterMethod=Forward Euler  ControllerParametersSource=internal  P=0.2  I=0  D=0.2  UseFilter=on  N=100  TunerSelectOption=Transfer Function Based (PID Tuner App)  InitialConditionSource=internal  InitialConditionForIntegrator=0  InitialConditionForFilter=0  DifferentiatorICPrevScaledInput=0  ExternalReset=none  TrackingMode=off  Kt=1  LimitOutput=off  SatLimitsSource=internal  UpperSaturationLimit=inf  LowerSaturationLimit=-inf  LinearizeAsGain=on  AntiWindupMode=none  Kb=1  POutMin=[]  POutMax=[]  IOutMin=[]  IOutMax=[]  DOutMin=[]  DOutMax=[]  NOutMin=[]  NOutMax=[]  SumOutMin=[]  SumOutMax=[]  SaturationOutMin=[]  SaturationOutMax=[]  PParamMin=[]  PParamMax=[]  IParamMin=[]  IParamMax=[]  DParamMin=[]  DParamMax=[]  NParamMin=[]  NParamMax=[]  KbParamMin=[]  KbParamMax=[]  KtParamMin=[]  KtParamMax=[]  KbOutMin=[]  KbOutMax=[]  KtOutMin=[]  KtOutMax=[]  IntegratorOutMin=[]  IntegratorOutMax=[]  FilterOutMin=[]  FilterOutMax=[]  SumI1OutMin=[]  SumI1OutMax=[]  SumI2OutMin=[]  SumI2OutMax=[]  SumI3OutMin=[]  SumI3OutMax=[]  SumI4OutMin=[]  SumI4OutMax=[]  SumDOutMin=[]  SumDOutMax=[]  DifferentiatorOutMin=[]  DifferentiatorOutMax=[]  FilterDiffOutCoefMin=[]  FilterDiffOutCoefMax=[]  ReciprocalOutMin=[]  ReciprocalOutMax=[]  SumDenOutMin=[]  SumDenOutMax=[]  SumNumOutMin=[]  SumNumOutMax=[]  DivideOutMin=[]  DivideOutMax=[]  UdiffTsProdOutMin=[]  UdiffTsProdOutMax=[]  NTsProdOutMin=[]  NTsProdOutMax=[]  UintegralTsProdOutMin=[]  UintegralTsProdOutMax=[]  UngainTsProdOutMin=[]  UngainTsProdOutMax=[]  IntegratorContinuousStateAttributes=''  IntegratorStateMustResolveToSignalObject=off  IntegratorRTWStateStorageClass=Auto  FilterContinuousStateAttributes=''  FilterStateMustResolveToSignalObject=off  FilterRTWStateStorageClass=Auto  ParallelPVariant=InternalParameters  IdealPVariant=Disabled  IVariant=InternalParameters  DVariant=InternalParameters  IntegratorVariant=Continuous  SatVariant=Disabled  AWVariant=Passthrough  PCopyVariant=Disabled  TRVariant=Disabled  FdbkBlocksVariant=Forward  IdealPFdbkVariant=Disabled  SatFdbkVariant=Disabled  DerivativeFilterVariant=ContFilter  NVariant=InternalParameters  NCopyVariant=Disabled  FilterICVariant=InternalICsFilter  IntegratorICVariant=InternalICs  ExternalResetVariant=Disabled  TRSumVariant=Passthrough  SumFdbkVariant=Disabled  SumVariant=Sum_PID  TsampFilterVariant=InternalTs  TsampNgainVariant=Passthrough  TsampIntegralVariant=Passthrough  ExternalSaturationOutDataTypeStr=Inherit: Same as second input
  Saturation TN : Saturate  UpperLimit=1  LowerLimit=-1
  Saturation TX : Saturate  UpperLimit=1  LowerLimit=-1
  Saturation TZ : Saturate  UpperLimit=1  LowerLimit=-1
  Sum : Sum  Inputs=|+-
  Switch : Switch  Criteria=u2 > Threshold
  Switch1 : Switch  Criteria=u2 > Threshold
  Unwrap : Subsystem
  Tin : Outport  VectorParamsAs1DForOutWhenUnconnected=off
  Actuators Choice O : Outport  Port=2  VectorParamsAs1DForOutWhenUnconnected=off
  wires:
  Mux/1 -> Tin/1  "[TX TN TZ]"
  Saturation TZ/1 -> Mux/3  "TZ"
  Saturation TX/1 -> Mux/1  "TX"
  In Bus Element4/1 -> PID Controller TZ Phin/1, PID Controller TZ Prop/1
  In Bus Element3/1 -> Sum/1  "Yaw_d"
  Saturation TN/1 -> Mux/2  "TN"
  In Bus Element2/1 -> PID Controller TX Phin/1, PID Controller TX Prop/1
  PID Controller TN/1 -> Saturation TN/1
  In Bus Element/1 -> Actuators Choice O/1, Switch/2
  Switch/1 -> Saturation TX/1
  PID Controller TX Prop/1 -> Switch/1
  PID Controller TX Phin/1 -> Switch/3
  In Bus Element1/1 -> Unwrap/1(yaw in)
  Unwrap/1(yaw out) -> Sum/2  "Yaw"
  Sum/1 -> PID Controller TN/1
  Switch1/1 -> Saturation TZ/1
  In Bus Element5/1 -> Switch1/2
  PID Controller TZ Prop/1 -> Switch1/1
  PID Controller TZ Phin/1 -> Switch1/3

== system RoboticFish_NGC/Guidance and Control system/ Guidance system/Distance ==
  "[Xe Ye]" : Inport
  Demux : Demux  Outputs=2
  Plus : Sum
  Sqrt : Sqrt  SaturateOnIntegerOverflow=on
  Square : Math  Operator=square  SignedPower=on  SaturateOnIntegerOverflow=on
  Square1 : Math  Operator=square  SignedPower=on  SaturateOnIntegerOverflow=on
  D : Outport  VectorParamsAs1DForOutWhenUnconnected=off
  wires:
  Demux/2 -> Square1/1  "Y"
  Square/1 -> Plus/1  "X^2"
  Square1/1 -> Plus/2  "Y^2"
  Plus/1 -> Sqrt/1  "X^2 + Y^2"
  Sqrt/1 -> D/1  "sqrt(X^2 + Y^2 )"
  Demux/1 -> Square/1  "X"
  "[Xe Ye]"/1 -> Demux/1

== system RoboticFish_NGC/Guidance and Control system/ Guidance system/LOS law ==
  "[Xe Ye]" : Inport
  Atan2 : Trigonometry  Operator=atan2
  Gain3 : Gain  Gain=180/pi
  Selector : Selector  InputPortWidth=2  IndexOptions=Index vector (dialog)  Indices=[2]  OutputSizes=1
  Selector3 : Selector  InputPortWidth=2  IndexOptions=Index vector (dialog)  Indices=[1]  OutputSizes=1
  "Unwrap " : dspsigops/Unwrap  tol=pi  InputProcessing=Columns as channels (frame based)  running=off
  Yaw_d : Outport  VectorParamsAs1DForOutWhenUnconnected=off
  wires:
  Selector/1 -> Atan2/1  "Ye"
  Selector3/1 -> Atan2/2  "Xe"
  "[Xe Ye]"/1 -> Selector3/1, Selector/1
  Gain3/1 -> Yaw_d/1
  Atan2/1 -> "Unwrap "/1
  "Unwrap "/1 -> Gain3/1

== system RoboticFish_NGC/Robotic-Fish Model & PropulsionSystem/Propulsion System/Horizontal Force and Moment (Tau_H) ==
  note: calcolo modulo: U=modulo(u v w)
  uHT3 : Inport
  uHT1 : Inport  Port=2
  uHT2 : Inport  Port=3
  nu_B : Inport  Port=4
  Dot Product : DotProduct  InputSameDT=on  OutDataTypeStr=Inherit: Inherit via internal rule
  HT_prop : Constant  Value=HT_prop
  Matrix Multiply : Product  Multiplication=Matrix(*)
  Mux : Mux  Inputs=3
  Mux1 : Mux  Inputs=2
  Selector : Selector  InputPortWidth=6  IndexOptions=Index vector (dialog)  Indices=[1 2 3]  OutputSizes=1
  Sqrt : Sqrt  SaturateOnIntegerOverflow=on
  Sum : Sum  Inputs=|++
  Tau_HT3 (Tau_Caudal_Fin) : Subsystem
  t : Clock
  Horizontal _Tau : Outport  VectorParamsAs1DForOutWhenUnconnected=off
  wires:
  uHT1/1 -> Mux1/1
  Tau_HT3 (Tau_Caudal_Fin)/1(Tau_HT3) -> Sum/1  "[Tau_surge_HT3 Tau_sway_HT3 0 0 0 Tau_yaw_HT3]"
  uHT2/1 -> Mux1/2
  Matrix Multiply/1 -> Sum/2  "[surge_HT1&HT2 0 0 0 0 yaw_HT1&HT2]"
  Mux1/1 -> Matrix Multiply/2
  HT_prop/1 -> Matrix Multiply/1
  Sum/1 -> Horizontal _Tau/1  "Tau_HT3+Tau_HT1&HT2"
  nu_B/1 -> Selector/1
  Selector/1 -> Dot Product/1, Dot Product/2
  Mux/1 -> Tau_HT3 (Tau_Caudal_Fin)/1("[U uHT3 t]")
  t/1 -> Mux/3
  Dot Product/1 -> Sqrt/1
  uHT3/1 -> Mux/2  "[f_%  Thetastr_%]"
  Sqrt/1 -> Mux/1  "U"

== system RoboticFish_NGC/Robotic-Fish Model & PropulsionSystem/Propulsion System/Subsystem ==
  D_uVT2  D_uVT3 : Inport
  uCMD : Inport  Port=2
  Bus Creator : BusCreator  Inputs=7
  Bus Selector : BusSelector  OutputSignals=D_VT2,D_VT3
  Bus Selector1 : BusSelector  OutputSignals=f_HT3,Thetastr_HT3,uHT1,uHT2,uVT1
  "ucmd " : Outport  VectorParamsAs1DForOutWhenUnconnected=off
  wires:
  D_uVT2  D_uVT3/1 -> Bus Selector/1
  uCMD/1 -> Bus Selector1/1
  Bus Selector/1 -> Bus Creator/6  "<D_VT2>"
  Bus Selector/2 -> Bus Creator/7  "<D_VT3>"
  Bus Selector1/5 -> Bus Creator/5  "<uVT1>"
  Bus Selector1/4 -> Bus Creator/4  "<uHT2>"
  Bus Selector1/3 -> Bus Creator/3  "<uHT1>"
  Bus Selector1/2 -> Bus Creator/2  "<Thetastr_HT3>"
  Bus Selector1/1 -> Bus Creator/1  "<f_HT3>"
  Bus Creator/1 -> "ucmd "/1
